simulink model "controlador_integrador_LPV"  (R2018b)
settings: Solver=FixedStepAuto  StartTime=0.0  StopTime=3000  FixedStep=T  RelTol=1e-3
values from neighbouring files (symbols this model uses):
  T = 5.2632    [termos_de_Ad.m]
undefined symbols (not defined in the file or in its folder): DiscIntNeverNeededParam
settings Model: Creator=tarsis  LastModifiedBy=tarsis

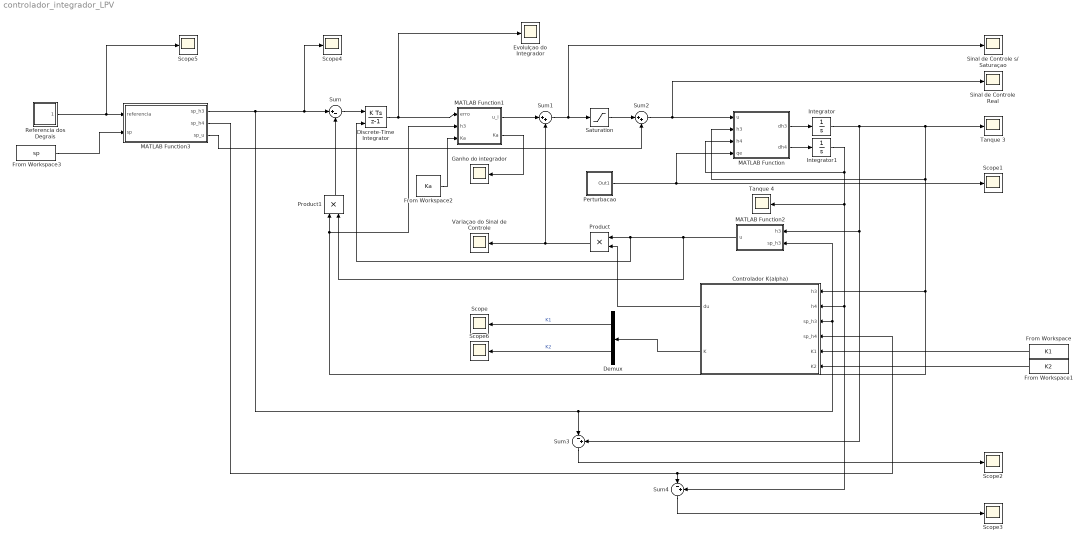
== system controlador_integrador_LPV ==
  Controlador K(alpha) : MATLAB Function  TreatAsAtomicUnit=on
  Demux : Demux  Outputs=2
  Discrete-Time Integrator : DiscreteIntegrator  gainval=1/T  ExternalReset=rising  SampleTime=T  ICPrevOutput=DiscIntNeverNeededParam  ICPrevScaledInput=DiscIntNeverNeededParam
  Evolulçao do Integrador : Scope
  From Workspace : FromWorkspace  VariableName=K1  SampleTime=0
  From Workspace1 : FromWorkspace  VariableName=K2  SampleTime=0
  From Workspace2 : FromWorkspace  VariableName=Ka  SampleTime=0
  From Workspace3 : FromWorkspace  VariableName=sp  SampleTime=T
  Ganho do integrador : Scope
  Integrator : Integrator
  Integrator1 : Integrator
  MATLAB Function : MATLAB Function  TreatAsAtomicUnit=on
  MATLAB Function1 : MATLAB Function  TreatAsAtomicUnit=on
  MATLAB Function2 : MATLAB Function  TreatAsAtomicUnit=on
  MATLAB Function3 : MATLAB Function  TreatAsAtomicUnit=on
  Perturbacao : Subsystem
  Product : Product
  Product1 : Product
  Referencia dos Degrais : Subsystem
  Saturation : Saturate  UpperLimit=15  LowerLimit=-15
  Scope{,1..6} (7 alike) : Scope
  Sinal de Controle Real : Scope
  Sinal de Controle s/ Saturaçao : Scope
  Sum : Sum  Inputs=|+-
  Sum1 : Sum  Inputs=|++
  Sum2 : Sum  Inputs=|++
  Sum3 : Sum  Inputs=|-+
  Sum4 : Sum  Inputs=|-+
  Tanque 3 : Scope
  Tanque 4 : Scope
  "Variaçao do Sinal de Controle " : Scope
  wires:
  MATLAB Function2/1(u) -> Discrete-Time Integrator/2, Product/1, Product1/2
  Product/1 -> "Variaçao do Sinal de Controle "/1, Sum1/2
  MATLAB Function/1(dh3) -> Integrator/1
  Controlador K(alpha)/1(du) -> Product/2
  Integrator1/1 -> Sum4/2, Controlador K(alpha)/2(h4), Tanque 4/1, MATLAB Function/3(h4)
  Demux/2 -> Scope6/1  "K2"
  Demux/1 -> Scope/1  "K1"
  Controlador K(alpha)/2(K) -> Demux/1
  MATLAB Function/2(dh4) -> Integrator1/1
  Integrator/1 -> Tanque 3/1, Product1/1, MATLAB Function1/2(h3), Controlador K(alpha)/1(h3), MATLAB Function/2(h3), Sum3/2, MATLAB Function2/1(h3)
  MATLAB Function1/1(u_i) -> Sum1/1
  Sum1/1 -> Saturation/1, Sinal de Controle s/ Saturaçao/1
  Product1/1 -> Sum/2
  Sum/1 -> Discrete-Time Integrator/1
  Discrete-Time Integrator/1 -> Evolulçao do Integrador/1, MATLAB Function1/1(erro)
  MATLAB Function1/2(Ka) -> Ganho do integrador/1
  Perturbacao/1(Out1) -> Scope1/1, MATLAB Function/4(qe)
  Sum2/1 -> Sinal de Controle Real/1, MATLAB Function/1(u)
  Saturation/1 -> Sum2/1
  Sum3/1 -> Scope2/1
  Sum4/1 -> Scope3/1
  Referencia dos Degrais/1(Out1) -> Scope5/1, MATLAB Function3/1(referencia)
  From Workspace/1 -> Controlador K(alpha)/5(K1)
  From Workspace1/1 -> Controlador K(alpha)/6(K2)
  From Workspace2/1 -> MATLAB Function1/3("Ka ")
  MATLAB Function3/1(sp_h3) -> Sum3/1, Controlador K(alpha)/3(sp_h3), MATLAB Function2/2(sp_h3), Scope4/1, Sum/1
  MATLAB Function3/2(sp_h4) -> Sum4/1, Controlador K(alpha)/4(sp_h4)
  MATLAB Function3/3(sp_u) -> Sum2/2
  From Workspace3/1 -> MATLAB Function3/2(sp)

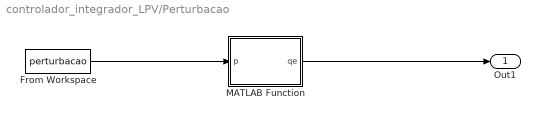
== system controlador_integrador_LPV/Perturbacao ==
  From Workspace : FromWorkspace  VariableName=perturbacao  SampleTime=T  OutputAfterFinalValue=Setting to zero
  MATLAB Function : MATLAB Function  TreatAsAtomicUnit=on
  Out1 : Outport
  wires:
  From Workspace/1 -> MATLAB Function/1(p)
  MATLAB Function/1(qe) -> Out1/1

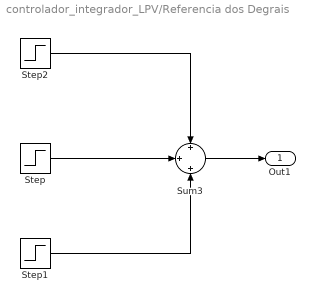
== system controlador_integrador_LPV/Referencia dos Degrais ==
  Step : Step  Time=1000  After=0.02  SampleTime=T
  Step1 : Step  Time=2000  After=0.02  SampleTime=T
  Step2 : Step  Time=0  After=0.28  SampleTime=T
  Sum3 : Sum  Inputs=+|+|+
  Out1 : Outport
  wires:
  Step/1 -> Sum3/2
  Sum3/1 -> Out1/1
  Step2/1 -> Sum3/1
  Step1/1 -> Sum3/3

== matlab function controlador_integrador_LPV/Controlador K(alpha) ==
  data: h3 input; du output; h4 input; sp_h3 input; sp_h4 input; K output; K1 input; K2 input
function [du,K] = fcn(h3,h4,sp_h3,sp_h4,K1,K2)
h = [h4 h3]';
sp_h = [sp_h4 sp_h3]';

K = h3*0.05*(K2 - K1) + 2.4*K1 - 1.4*K2;
du = K*(h - sp_h);

== matlab function controlador_integrador_LPV/MATLAB Function ==
  data: u input; dh3 output; dh4 output; h3 input; h4 input; qe input
function [dh3,dh4] = fcn(u,h3,h4,qe)
qi = (16.4*u + 357.3)*1e-6;
q12 = 33.51e-4*(h4 - h3) + 43.12e-5;
qout = (87.07e-5*sqrt(h3) + 30.99e-5);
A1 = (pi*(31)^2)*1e-4;
A2 = - 0.88629272879272778105782609278436*h3^16 + 6.0267905557905489111932174309337*h3^15 - 20.80464391736738395516887057851*h3^14 + 47.68494439008527766774004035511*h3^13 - 82.573907447205791291786792565001*h3^12 + 116.28257881925208875326233578017*h3^11 - 139.30893428077013388311346843447*h3^10 + 144.80767028205944702410747888441*h3^9 - 129.2475129476872169884635810807*h3^8 + 96.099152680911332924853135955618*h3^7 - 55.593870964701796673125553833866*h3^6 + 21.451550218200266654046211819752*h3^5 - 5.9275208717979510465216954484015*h3^4 + 3.9856416105248966168880953176109*h3^3 - 2.0902185091906828919771687989635*h3^2 - 0.061481774188906647716430580264178*h3 + 0.32722421068834535751546101783638;
dh4 = (qi - q12)/A1;
dh3 = (q12 - qout + qe)/A2;

== matlab function controlador_integrador_LPV/MATLAB Function2 ==
  settings: updateMethod=DISCRETE
  data: h3 input; u output; sp_h3 input
function u = fcn(h3,sp_h3)

persistent s
if isempty(s)
    s = false;
end

if h3<sp_h3*0.95 && s==false
    u = 0;
else
    u = 1;
    s = true;
end

== matlab function controlador_integrador_LPV/MATLAB Function1 ==
  data: erro input; u_i output; h3 input; Ka output; Ka input
function [u_i,Ka] = fcn(erro,h3,Ka)
Ka1 = Ka(1);
Ka2 = Ka(2);
Ka = h3*0.05*(Ka1 -Ka2) + 2.4*Ka1 - 1.4*Ka2;
u_i = Ka*erro;

== matlab function controlador_integrador_LPV/MATLAB Function3 ==
  data: sp_h3 output; sp_h4 output; referencia input; sp_u output; sp input
function [sp_h3,sp_h4,sp_u] = fcn(referencia,sp)
if referencia == sp.h3(1)
    sp_u = sp.u(1);
    sp_h3 = sp.h3(1);
    sp_h4 = sp.h4(1);
elseif referencia > sp.h3(1) && referencia < sp.h3(2)
    sp_u = sp.u(2);
    sp_h3 = sp.h3(2);
    sp_h4 = sp.h4(2);
else
    sp_u = sp.u(3);
    sp_h3 = sp.h3(3);
    sp_h4 = sp.h4(3);
end

== matlab function controlador_integrador_LPV/Perturbacao/MATLAB Function ==
  data: p input; qe output
function qe = fcn(p)
persistent d
if isempty(d)
    d = 1;
end
if (d < 138)
    d = d +1; 
    qe = 0;
else
%     qe = ((2.35e-2)^2)*(pi/4)*sqrt(2*9.80655*p);
    qe = 0;
end
